simulink model "Position_Motor_Controller_v3"  (R2018b)
settings: Solver=VariableStepAuto  StartTime=0.0  StopTime=10.0  RelTol=1e-3
libraries: simulink x3
settings Model: Creator=James  LastModifiedBy=james.quan.166

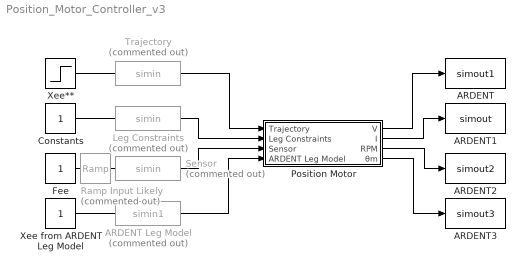
== system Position_Motor_Controller_v3 ==
  ARDENT : ToWorkspace  VariableName=simout1  SaveFormat=Timeseries  SampleTime=-1
  ARDENT Leg Model : FromWorkspace  Commented=on  VariableName=simin1  SampleTime=0
  ARDENT1 : ToWorkspace  VariableName=simout  SaveFormat=Timeseries  SampleTime=-1
  ARDENT2 : ToWorkspace  VariableName=simout2  SaveFormat=Timeseries  SampleTime=-1
  ARDENT3 : ToWorkspace  VariableName=simout3  SaveFormat=Timeseries  SampleTime=-1
  Constants : Constant
  Fee : Constant
  Leg Constraints : FromWorkspace  Commented=on  VariableName=simin  SampleTime=0
  Position Motor : Subsystem
  Ramp Input Likely : simulink/Sources/Ramp  Commented=on  slope=1  start=0  InitialOutput=0
  Sensor : FromWorkspace  Commented=on  VariableName=simin  SampleTime=0
  Trajectory : FromWorkspace  Commented=on  VariableName=simin  SampleTime=0
  Xee from ARDENT Leg Model : Constant
  Xee** : Step  After=10  SampleTime=0
  wires:
  Position Motor/1(V) -> ARDENT/1
  Position Motor/4(θm) -> ARDENT3/1
  Position Motor/3(RPM) -> ARDENT2/1
  Position Motor/2(I) -> ARDENT1/1
  Xee from ARDENT Leg Model/1 -> Position Motor/4(ARDENT Leg Model)
  Constants/1 -> Position Motor/2(Leg Constraints)
  Fee/1 -> Position Motor/3(Sensor)
  Xee**/1 -> Position Motor/1(Trajectory)

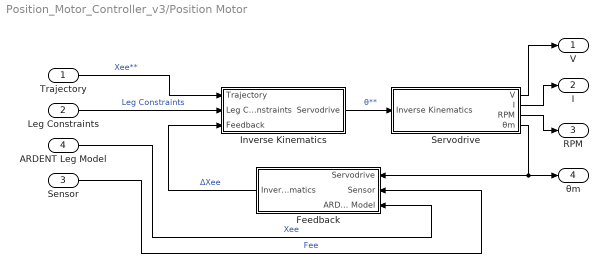
== system Position_Motor_Controller_v3/Position Motor ==
  Trajectory : Inport
  Leg Constraints : Inport  Port=2
  Sensor : Inport  Port=3
  ARDENT Leg Model : Inport  Port=4
  Feedback : Subsystem
  Inverse Kinematics : Subsystem
  Servodrive : Subsystem
  V : Outport
  I : Outport  Port=2
  RPM : Outport  Port=3
  θm : Outport  Port=4
  wires:
  Inverse Kinematics/1(Servodrive) -> Servodrive/1(Inverse Kinematics)  "θ**"
  Leg Constraints/1 -> Inverse Kinematics/2(Leg Constraints)  "Leg Constraints"
  Sensor/1 -> Feedback/2(Sensor)  "Fee"
  Feedback/1(Inverse Kinematics) -> Inverse Kinematics/3(Feedback)  "ΔXee"
  ARDENT Leg Model/1 -> Feedback/3(ARDENT Leg Model)  "Xee"
  Trajectory/1 -> Inverse Kinematics/1(Trajectory)  "Xee**"
  Servodrive/4(θm) -> Feedback/1(Servodrive), θm/1
  Servodrive/3(RPM) -> RPM/1
  Servodrive/2(I) -> I/1
  Servodrive/1(V) -> V/1

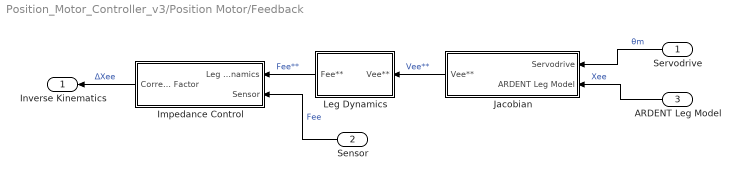
== system Position_Motor_Controller_v3/Position Motor/Feedback ==
  Servodrive : Inport
  Sensor : Inport  Port=2
  ARDENT Leg Model : Inport  Port=3
  Impedance Control : Subsystem
  Jacobian : Subsystem
  Leg Dynamics : Subsystem
  Inverse Kinematics : Outport
  wires:
  Impedance Control/1(Correction Factor) -> Inverse Kinematics/1  "ΔXee"
  Jacobian/1(Vee**) -> Leg Dynamics/1(Vee**)  "Vee**"
  Sensor/1 -> Impedance Control/2(Sensor)  "Fee"
  Leg Dynamics/1(Fee**) -> Impedance Control/1(Leg Dynamics)  "Fee**"
  ARDENT Leg Model/1 -> Jacobian/2(ARDENT Leg Model)  "Xee"
  Servodrive/1 -> Jacobian/1(Servodrive)  "θm"

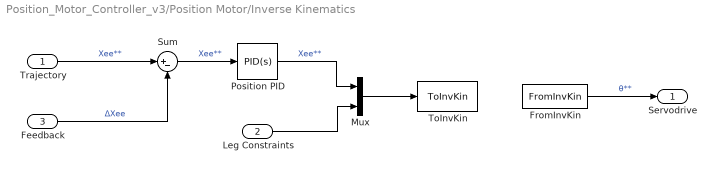
== system Position_Motor_Controller_v3/Position Motor/Inverse Kinematics ==
  Trajectory : Inport
  Leg Constraints : Inport  Port=2
  Feedback : Inport  Port=3
  FromInvKin : FromWorkspace  VariableName=FromInvKin  SampleTime=0
  Mux : Mux  Inputs=2
  Position PID : simulink/Continuous/PID Controller  Controller=PID  Form=Parallel  TimeDomain=Continuous-time  SampleTime=-1  IntegratorMethod=Forward Euler  FilterMethod=Forward Euler  ControllerParametersSource=internal  P=1  I=1  D=0  UseFilter=on  N=100  TunerSelectOption=Transfer Function Based (PID Tuner App)  InitialConditionSource=internal  InitialConditionForIntegrator=0  InitialConditionForFilter=0  DifferentiatorICPrevScaledInput=0  ExternalReset=none  TrackingMode=off  Kt=1  LimitOutput=off  UpperSaturationLimit=inf  LowerSaturationLimit=-inf  LinearizeAsGain=on  AntiWindupMode=none  Kb=1  POutMin=[]  POutMax=[]  IOutMin=[]  IOutMax=[]  DOutMin=[]  DOutMax=[]  NOutMin=[]  NOutMax=[]  SumOutMin=[]  SumOutMax=[]  SaturationOutMin=[]  SaturationOutMax=[]  PParamMin=[]  PParamMax=[]  IParamMin=[]  IParamMax=[]  DParamMin=[]  DParamMax=[]  NParamMin=[]  NParamMax=[]  KbParamMin=[]  KbParamMax=[]  KtParamMin=[]  KtParamMax=[]  KbOutMin=[]  KbOutMax=[]  KtOutMin=[]  KtOutMax=[]  IntegratorOutMin=[]  IntegratorOutMax=[]  FilterOutMin=[]  FilterOutMax=[]  SumI1OutMin=[]  SumI1OutMax=[]  SumI2OutMin=[]  SumI2OutMax=[]  SumI3OutMin=[]  SumI3OutMax=[]  SumI4OutMin=[]  SumI4OutMax=[]  SumDOutMin=[]  SumDOutMax=[]  DifferentiatorOutMin=[]  DifferentiatorOutMax=[]  FilterDiffOutCoefMin=[]  FilterDiffOutCoefMax=[]  ReciprocalOutMin=[]  ReciprocalOutMax=[]  SumDenOutMin=[]  SumDenOutMax=[]  SumNumOutMin=[]  SumNumOutMax=[]  DivideOutMin=[]  DivideOutMax=[]  IntegratorContinuousStateAttributes=''  IntegratorStateMustResolveToSignalObject=off  IntegratorRTWStateStorageClass=Auto  FilterContinuousStateAttributes=''  FilterStateMustResolveToSignalObject=off  FilterRTWStateStorageClass=Auto  ParallelPVariant=InternalParameters  IdealPVariant=Disabled  IVariant=InternalParameters  DVariant=InternalParameters  IntegratorVariant=Continuous  SatVariant=Disabled  AWVariant=Passthrough  PCopyVariant=Disabled  TRVariant=Disabled  FdbkBlocksVariant=Forward  IdealPFdbkVariant=Disabled  SatFdbkVariant=Disabled  DerivativeFilterVariant=ContFilter  NVariant=InternalParameters  NCopyVariant=Disabled  FilterICVariant=InternalICsFilter  IntegratorICVariant=InternalICs  ExternalResetVariant=Disabled  TRSumVariant=Passthrough  SumFdbkVariant=Disabled  SumVariant=Sum_PID
  Sum : Sum  Inputs=|+-
  ToInvKin : ToWorkspace  VariableName=ToInvKin  SaveFormat=Timeseries  SampleTime=-1
  Servodrive : Outport
  wires:
  Trajectory/1 -> Sum/1  "Xee**"
  Leg Constraints/1 -> Mux/2
  Feedback/1 -> Sum/2  "ΔXee"
  Mux/1 -> ToInvKin/1
  FromInvKin/1 -> Servodrive/1  "θ**"
  Sum/1 -> Position PID/1  "Xee**"
  Position PID/1 -> Mux/1  "Xee**"

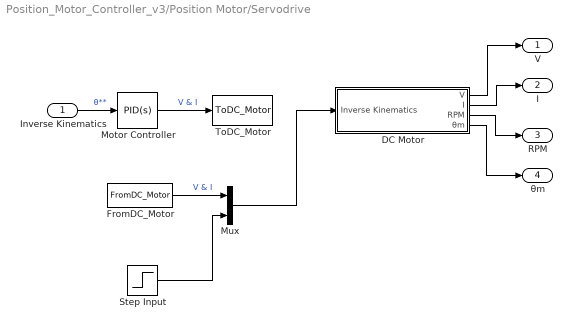
== system Position_Motor_Controller_v3/Position Motor/Servodrive ==
  Inverse Kinematics : Inport
  DC Motor : Subsystem
  FromDC_Motor : FromWorkspace  VariableName=FromDC_Motor  SampleTime=0
  Motor Controller : simulink/Continuous/PID Controller  Controller=PID  Form=Parallel  TimeDomain=Continuous-time  SampleTime=-1  IntegratorMethod=Forward Euler  FilterMethod=Forward Euler  ControllerParametersSource=internal  P=1  I=1  D=0  UseFilter=on  N=100  TunerSelectOption=Transfer Function Based (PID Tuner App)  InitialConditionSource=internal  InitialConditionForIntegrator=0  InitialConditionForFilter=0  DifferentiatorICPrevScaledInput=0  ExternalReset=none  TrackingMode=off  Kt=1  LimitOutput=off  UpperSaturationLimit=inf  LowerSaturationLimit=-inf  LinearizeAsGain=on  AntiWindupMode=none  Kb=1  POutMin=[]  POutMax=[]  IOutMin=[]  IOutMax=[]  DOutMin=[]  DOutMax=[]  NOutMin=[]  NOutMax=[]  SumOutMin=[]  SumOutMax=[]  SaturationOutMin=[]  SaturationOutMax=[]  PParamMin=[]  PParamMax=[]  IParamMin=[]  IParamMax=[]  DParamMin=[]  DParamMax=[]  NParamMin=[]  NParamMax=[]  KbParamMin=[]  KbParamMax=[]  KtParamMin=[]  KtParamMax=[]  KbOutMin=[]  KbOutMax=[]  KtOutMin=[]  KtOutMax=[]  IntegratorOutMin=[]  IntegratorOutMax=[]  FilterOutMin=[]  FilterOutMax=[]  SumI1OutMin=[]  SumI1OutMax=[]  SumI2OutMin=[]  SumI2OutMax=[]  SumI3OutMin=[]  SumI3OutMax=[]  SumI4OutMin=[]  SumI4OutMax=[]  SumDOutMin=[]  SumDOutMax=[]  DifferentiatorOutMin=[]  DifferentiatorOutMax=[]  FilterDiffOutCoefMin=[]  FilterDiffOutCoefMax=[]  ReciprocalOutMin=[]  ReciprocalOutMax=[]  SumDenOutMin=[]  SumDenOutMax=[]  SumNumOutMin=[]  SumNumOutMax=[]  DivideOutMin=[]  DivideOutMax=[]  IntegratorContinuousStateAttributes=''  IntegratorStateMustResolveToSignalObject=off  IntegratorRTWStateStorageClass=Auto  FilterContinuousStateAttributes=''  FilterStateMustResolveToSignalObject=off  FilterRTWStateStorageClass=Auto  ParallelPVariant=InternalParameters  IdealPVariant=Disabled  IVariant=InternalParameters  DVariant=InternalParameters  IntegratorVariant=Continuous  SatVariant=Disabled  AWVariant=Passthrough  PCopyVariant=Disabled  TRVariant=Disabled  FdbkBlocksVariant=Forward  IdealPFdbkVariant=Disabled  SatFdbkVariant=Disabled  DerivativeFilterVariant=ContFilter  NVariant=InternalParameters  NCopyVariant=Disabled  FilterICVariant=InternalICsFilter  IntegratorICVariant=InternalICs  ExternalResetVariant=Disabled  TRSumVariant=Passthrough  SumFdbkVariant=Disabled  SumVariant=Sum_PID
  Mux : Mux  Inputs=2
  Step Input : Step  After=10  SampleTime=0
  ToDC_Motor : ToWorkspace  VariableName=ToDC_Motor  SaveFormat=Timeseries  SampleTime=-1
  V : Outport
  I : Outport  Port=2
  RPM : Outport  Port=3
  θm : Outport  Port=4
  wires:
  DC Motor/1(V) -> V/1
  Step Input/1 -> Mux/2
  FromDC_Motor/1 -> Mux/1  "V & I"
  Motor Controller/1 -> ToDC_Motor/1  "V & I"
  Inverse Kinematics/1 -> Motor Controller/1  "θ**"
  Mux/1 -> DC Motor/1(Inverse Kinematics)
  DC Motor/2(I) -> I/1
  DC Motor/3(RPM) -> RPM/1
  DC Motor/4(θm) -> θm/1

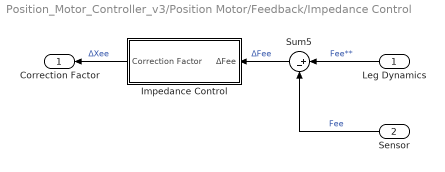
== system Position_Motor_Controller_v3/Position Motor/Feedback/Impedance Control ==
  Leg Dynamics : Inport
  Sensor : Inport  Port=2
  Impedance Control : Subsystem
  Sum5 : Sum  Inputs=|+-
  Correction Factor : Outport
  wires:
  Impedance Control/1(Correction Factor) -> Correction Factor/1  "ΔXee"
  Sum5/1 -> Impedance Control/1(ΔFee)  "ΔFee"
  Leg Dynamics/1 -> Sum5/1  "Fee**"
  Sensor/1 -> Sum5/2  "Fee"

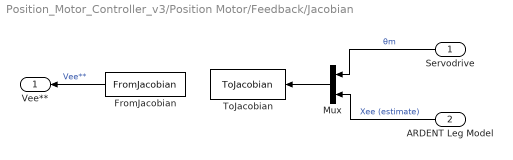
== system Position_Motor_Controller_v3/Position Motor/Feedback/Jacobian ==
  Servodrive : Inport
  ARDENT Leg Model : Inport  Port=2
  FromJacobian : FromWorkspace  VariableName=FromJacobian  SampleTime=0
  Mux : Mux  Inputs=2
  ToJacobian : ToWorkspace  VariableName=ToJacobian  SaveFormat=Timeseries  SampleTime=-1
  Vee** : Outport
  wires:
  Servodrive/1 -> Mux/1  "θm"
  ARDENT Leg Model/1 -> Mux/2  "Xee (estimate)"
  FromJacobian/1 -> Vee**/1  "Vee**"
  Mux/1 -> ToJacobian/1

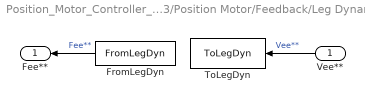
== system Position_Motor_Controller_v3/Position Motor/Feedback/Leg Dynamics ==
  Vee** : Inport
  FromLegDyn : FromWorkspace  VariableName=FromLegDyn  SampleTime=0
  ToLegDyn : ToWorkspace  VariableName=ToLegDyn  SaveFormat=Timeseries  SampleTime=-1
  Fee** : Outport
  wires:
  Vee**/1 -> ToLegDyn/1  "Vee**"
  FromLegDyn/1 -> Fee**/1  "Fee**"

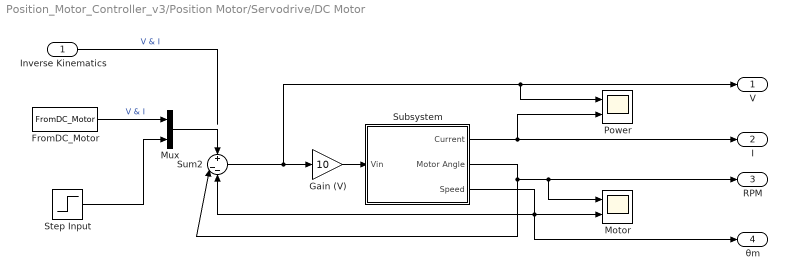
== system Position_Motor_Controller_v3/Position Motor/Servodrive/DC Motor ==
  Inverse Kinematics : Inport
  FromDC_Motor : FromWorkspace  VariableName=FromDC_Motor  SampleTime=0
  Gain (V) : Gain  Gain=10
  Motor : Scope  NumInputPorts=2
  Mux : Mux  Inputs=2
  Power : Scope  NumInputPorts=2
  Step Input : Step  After=10  SampleTime=0
  Subsystem : Subsystem
  Sum2 : Sum  Inputs=+|--
  V : Outport
  I : Outport  Port=2
  RPM : Outport  Port=3
  θm : Outport  Port=4
  wires:
  Inverse Kinematics/1 -> ?  "V & I"
  Step Input/1 -> Mux/2
  FromDC_Motor/1 -> Mux/1  "V & I"
  Subsystem/1(Current) -> I/1, Power/2
  Subsystem/2(Motor Angle) -> RPM/1, Motor/1, Sum2/2
  Mux/1 -> Sum2/1
  Subsystem/3(Speed) -> θm/1, Sum2/3, Motor/2
  Sum2/1 -> V/1, Power/1, Gain (V)/1
  Gain (V)/1 -> Subsystem/1(Vin)

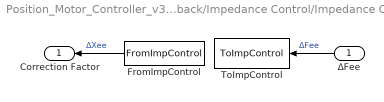
== system Position_Motor_Controller_v3/Position Motor/Feedback/Impedance Control/Impedance Control ==
  ΔFee : Inport
  FromImpControl : FromWorkspace  VariableName=FromImpControl  SampleTime=0
  ToImpControl : ToWorkspace  VariableName=ToImpControl  SaveFormat=Timeseries  SampleTime=-1
  Correction Factor : Outport
  wires:
  ΔFee/1 -> ToImpControl/1  "ΔFee"
  FromImpControl/1 -> Correction Factor/1  "ΔXee"

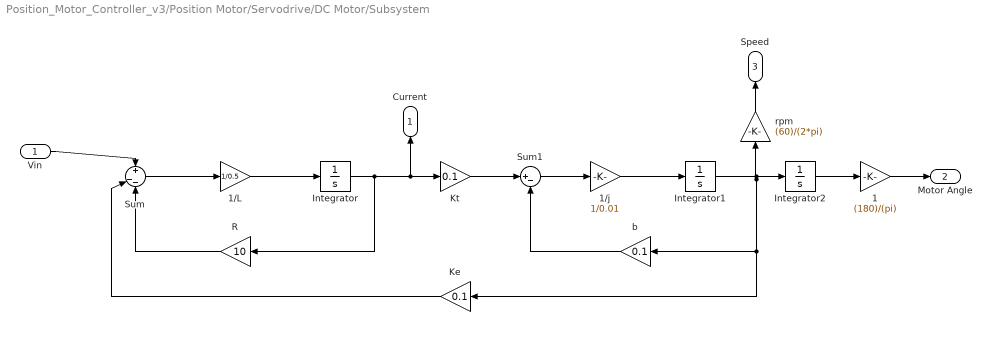
== system Position_Motor_Controller_v3/Position Motor/Servodrive/DC Motor/Subsystem ==
  Vin : Inport
  1 : Gain  Gain=(180)/(pi)
  1/L : Gain  Gain=1/0.5
  1/j : Gain  Gain=1/0.01
  Integrator : Integrator
  Integrator1 : Integrator
  Integrator2 : Integrator
  Ke : Gain  Gain=0.1
  "Kt " : Gain  Gain=0.1
  R : Gain  Gain=10
  Sum : Sum  Inputs=+|--
  Sum1 : Sum  Inputs=|+-
  "b " : Gain  Gain=0.1
  rpm : Gain  Gain=(60)/(2*pi)
  Current : Outport
  Motor Angle : Outport  Port=2
  Speed : Outport  Port=3
  wires:
  Integrator2/1 -> 1/1
  1/j/1 -> Integrator1/1
  "b "/1 -> Sum1/2
  1/L/1 -> Integrator/1
  Sum1/1 -> 1/j/1
  "Kt "/1 -> Sum1/1
  Sum/1 -> 1/L/1
  Integrator1/1 -> Integrator2/1, rpm/1, Ke/1, "b "/1
  Vin/1 -> Sum/1
  Ke/1 -> Sum/2
  R/1 -> Sum/3
  Integrator/1 -> Current/1, "Kt "/1, R/1
  rpm/1 -> Speed/1
  1/1 -> Motor Angle/1
